simulink model "GHV_open_VarialbeMass_toolbox_adaptive_fuzzy"  (R2023b)
settings: Solver=VariableStepAuto  StartTime=0.0  StopTime=130  FixedStep=0.0000001  MaxStep=0.001  RelTol=1e-3
InitFcn:
  | run('init.m')
undefined symbols (not defined in the file): GHV_cfg
libraries: aerolibasang x3, simulink_extras x2, shared6dof x1, aerolibadyn x1, aerolibatmos2 x1
settings Model: SimulationMode=accelerator  Creator=Admin  LastModifiedBy=Admin
settings SolverCC: AllowMultiTaskInputOutput=on  ZeroCrossControl=EnableAll  ZeroCrossAlgorithm=Adaptive  AutoInsertRateTranBlk=on
settings DebuggingCC: MaskedZcDiagnostic=none  IgnoredZcDiagnostic=none

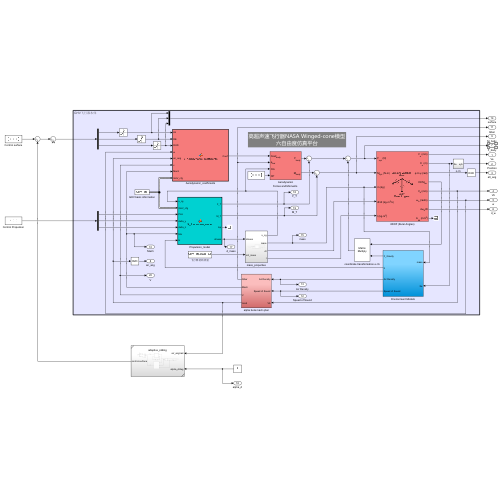
[thumbnail: Simulink's stored preview of the top-level diagram]
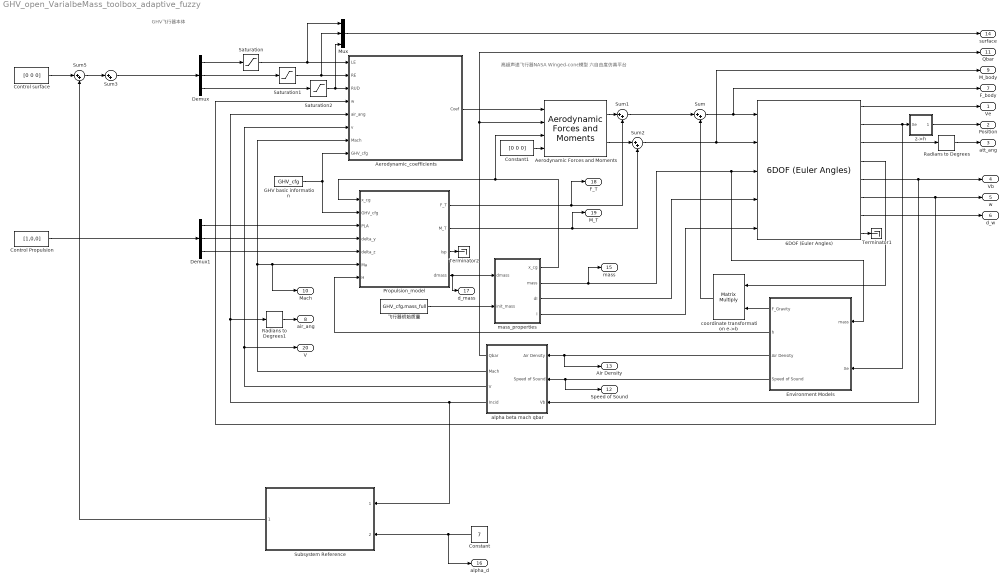
== system GHV_open_VarialbeMass_toolbox_adaptive_fuzzy ==
  note: GHV飞行器本体
  note: 高超声速飞行器NASA Winged-cone模型
      | 六自由度仿真平台
  6DOF (Euler Angles) : shared6dof/6DOF (Euler Angles)  units=Metric (MKS)  mtype=Custom Variable  rep=Euler Angles  xme_0=Position_init  Vm_0=Speed_init  eul_0=Euler_init  pm_0=Omega_init  mass_0=GHV_cfg.mass_full  mass_e=0.5  mass_f=2.0  inertia=GHV_cfg.J  inertia_e=eye(3)  inertia_f=2*eye(3)  k_quat=1.0  vre_flag=off  abi_flag=off  aMode=0  xme_statename=''  Vm_statename=''  eul_statename=''  quat_statename=''  pm_statename=''  mass_statename=''
  "Aerodynamic Forces and Moments " : aerolibadyn/Aerodynamic Forces and Moments   inputAxes=Body  outputForceAxes=Body  outputMomentAxes=Body  S=GHV_cfg.s_ref  b=GHV_cfg.b_ref  cbar=GHV_cfg.c_ref
  Aerodynamic_coefficients : MATLAB Function  TreatAsAtomicUnit=on
  Constant : Constant  Value=7
  Constant1 : Constant  Value=[0 0 0]
  Control Propulsion : Constant  Value=[1,0,0]
  Control surface : Constant  Value=[0 0 0]
  Demux : Demux  Outputs=3
  Demux1 : Demux  Outputs=3
  Environment Models : Subsystem
  GHV basic information : Constant  Value=GHV_cfg  VectorParams1D=off  OutDataTypeStr=Bus: slBus1
  Mux : Mux  Inputs=3
  Propulsion_model : MATLAB Function  TreatAsAtomicUnit=on
  Radians to Degrees : simulink_extras/Transformations/Radians to Degrees
  Radians to Degrees1 : simulink_extras/Transformations/Radians to Degrees
  Saturation : Saturate  UpperLimit=30  LowerLimit=-30
  Saturation1 : Saturate  UpperLimit=30  LowerLimit=-30
  Saturation2 : Saturate  UpperLimit=30  LowerLimit=-30
  Subsystem Reference : Subsystem  ReferencedSubsystem=adaptive_sliding
  Sum{,1..3,5} (5 alike) : Sum  Inputs=|++
  Terminator1 : Terminator
  Terminator2 : Terminator
  alpha beta mach qbar : Subsystem
  coordinate transformation e->b : Product  Multiplication=Matrix(*)
  mass_properties : Subsystem
  z->h : Subsystem
  飞行器初始质量 : Constant  Value=GHV_cfg.mass_full
  Ve : Outport
  Position : Outport  Port=2
  att_ang : Outport  Port=3
  Vb : Outport  Port=4
  w : Outport  Port=5
  d_w : Outport  Port=6
  F_body : Outport  Port=7
  air_ang : Outport  Port=8
  M_body : Outport  Port=9
  Mach : Outport  Port=10
  Qbar : Outport  Port=11
  Speed of Sound : Outport  Port=12
  Air Density : Outport  Port=13
  surface : Outport  Port=14
  mass : Outport  Port=15
  alpha_d : Outport  Port=16
  d_mass : Outport  Port=17
  F_T : Outport  Port=18
  M_T : Outport  Port=19
  V : Outport  Port=20
  wires:
  "Aerodynamic Forces and Moments "/1 -> Sum1/1
  "Aerodynamic Forces and Moments "/2 -> Sum2/1
  Aerodynamic_coefficients/1(Coef) -> "Aerodynamic Forces and Moments "/1
  Environment Models/1(F_Gravity) -> coordinate transformation e->b/2
  6DOF (Euler Angles)/4 -> coordinate transformation e->b/1
  Sum/1 -> 6DOF (Euler Angles)/1, F_body/1
  coordinate transformation e->b/1 -> Sum/2
  6DOF (Euler Angles)/2 -> z->h/1(Xe), Environment Models/2(Xe)
  Environment Models/4(Speed of Sound) -> Speed of Sound/1, alpha beta mach qbar/2(Speed of Sound)
  Environment Models/3(Air Density) -> Air Density/1, alpha beta mach qbar/1(Air Density)
  6DOF (Euler Angles)/5 -> Vb/1, alpha beta mach qbar/3(Vb)
  alpha beta mach qbar/1(Qbar) -> Qbar/1, "Aerodynamic Forces and Moments "/2
  alpha beta mach qbar/4(Incid) -> Subsystem Reference/1, Aerodynamic_coefficients/5(air_ang), Radians to Degrees1/1
  alpha beta mach qbar/3(V) -> V/1, Aerodynamic_coefficients/6(v)
  alpha beta mach qbar/2(Mach) -> Propulsion_model/6(Ma), Mach/1, Aerodynamic_coefficients/7(Mach)
  Constant1/1 -> "Aerodynamic Forces and Moments "/4
  6DOF (Euler Angles)/1 -> Ve/1
  6DOF (Euler Angles)/3 -> Radians to Degrees/1
  6DOF (Euler Angles)/7 -> d_w/1
  6DOF (Euler Angles)/8 -> Terminator1/1
  Control surface/1 -> Sum5/1
  GHV basic information/1 -> Propulsion_model/2(GHV_cfg), Aerodynamic_coefficients/8(GHV_cfg)
  z->h/1(xyh) -> Position/1
  Radians to Degrees/1 -> att_ang/1
  Radians to Degrees1/1 -> air_ang/1
  Demux/3 -> Saturation2/1
  6DOF (Euler Angles)/6 -> w/1, Aerodynamic_coefficients/4(w)
  Saturation/1 -> Mux/1, Aerodynamic_coefficients/1(LE)
  Saturation1/1 -> Mux/2, Aerodynamic_coefficients/2(RE)
  Saturation2/1 -> Mux/3, Aerodynamic_coefficients/3(RUD)
  Environment Models/2(h) -> Propulsion_model/7(H)
  Control Propulsion/1 -> Demux1/1
  Demux1/1 -> Propulsion_model/3(PLA)
  Demux1/3 -> Propulsion_model/5(delta_z)
  Demux1/2 -> Propulsion_model/4(delta_y)
  飞行器初始质量/1 -> mass_properties/2(init_mass)
  Propulsion_model/4(dmass) -> mass_properties/1(dmass), d_mass/1
  mass_properties/2(mass) -> mass/1, Environment Models/1(mass), 6DOF (Euler Angles)/3
  mass_properties/3(dI) -> 6DOF (Euler Angles)/4
  mass_properties/4(I) -> 6DOF (Euler Angles)/5
  mass_properties/1(x_cg) -> Propulsion_model/1(x_cg), "Aerodynamic Forces and Moments "/3
  Sum1/1 -> Sum/1
  Sum2/1 -> 6DOF (Euler Angles)/2, M_body/1
  Propulsion_model/1(F_T) -> F_T/1, Sum1/2
  Propulsion_model/2(M_T) -> M_T/1, Sum2/2
  Propulsion_model/3(Isp) -> Terminator2/1
  Mux/1 -> surface/1
  Constant/1 -> Subsystem Reference/2, alpha_d/1
  Demux/2 -> Saturation1/1
  Demux/1 -> Saturation/1
  Sum5/1 -> Sum3/1
  Subsystem Reference/1 -> Sum5/2
  Sum3/1 -> Demux/1

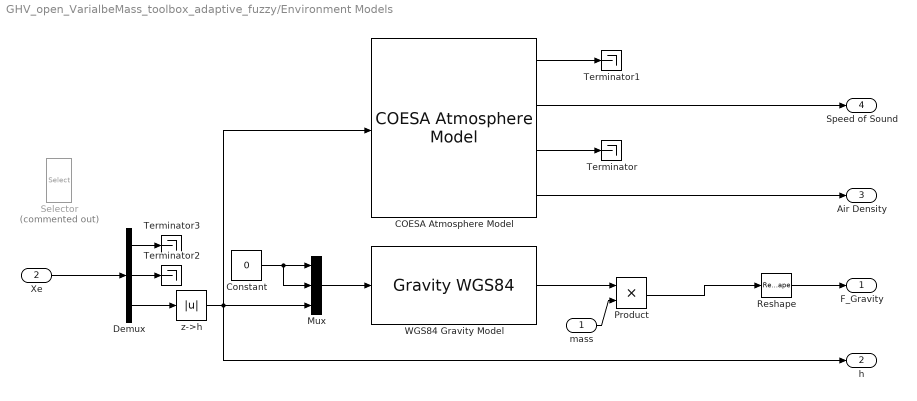
== system GHV_open_VarialbeMass_toolbox_adaptive_fuzzy/Environment Models ==
  mass : Inport
  Xe : Inport  Port=2
  COESA Atmosphere Model : aerolibatmos2/COESA Atmosphere Model  units=Metric (MKS)  spec=1976 COESA-extended U.S. Standard Atmosphere  model=Profile  profile_var=High temperature  profile_percent=1%  profile_alt=5 km (16404 ft)  envelope_var=High temperature  envelope_percent=1%  action=Warning
  Constant : Constant  Value=0
  Demux : Demux  Outputs=3
  Mux : Mux  Inputs=3
  Product : Product
  Reshape : Reshape
  Selector : Selector  Commented=on  InputPortWidth=3  IndexOptions=Index vector (dialog)  Indices=[3]  OutputSizes=1
  Terminator{,1..3} (4 alike) : Terminator
  "WGS84 Gravity Model  " : GravityWGS84  action=None
  z->h : Abs  SaturateOnIntegerOverflow=off
  F_Gravity : Outport
  h : Outport  Port=2
  Air Density : Outport  Port=3
  Speed of Sound : Outport  Port=4
  wires:
  Product/1 -> Reshape/1
  Constant/1 -> Mux/2, Mux/1
  z->h/1 -> h/1, COESA Atmosphere Model/1, Mux/3
  Mux/1 -> "WGS84 Gravity Model  "/1
  COESA Atmosphere Model/1 -> Terminator1/1
  COESA Atmosphere Model/2 -> Speed of Sound/1
  COESA Atmosphere Model/3 -> Terminator/1
  "WGS84 Gravity Model  "/1 -> Product/1
  COESA Atmosphere Model/4 -> Air Density/1
  Reshape/1 -> F_Gravity/1
  Xe/1 -> Demux/1
  Demux/3 -> z->h/1
  Demux/2 -> Terminator2/1
  Demux/1 -> Terminator3/1
  mass/1 -> Product/2

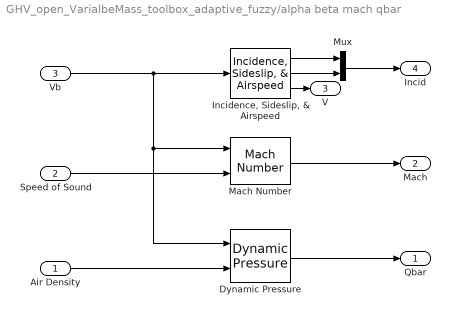
== system GHV_open_VarialbeMass_toolbox_adaptive_fuzzy/alpha beta mach qbar ==
  Air Density : Inport
  Speed of Sound : Inport  Port=2
  Vb : Inport  Port=3
  Dynamic Pressure : aerolibasang/Dynamic Pressure
  "Incidence, Sideslip, & Airspeed" : aerolibasang/Incidence, Sideslip, & Airspeed
  Mach Number : aerolibasang/Mach Number
  Mux : Mux  Inputs=2
  Qbar : Outport
  Mach : Outport  Port=2
  V : Outport  Port=3
  Incid : Outport  Port=4
  wires:
  Speed of Sound/1 -> Mach Number/2
  Mach Number/1 -> Mach/1
  "Incidence, Sideslip, & Airspeed"/2 -> Mux/2
  Vb/1 -> Dynamic Pressure/1, Mach Number/1, "Incidence, Sideslip, & Airspeed"/1
  Dynamic Pressure/1 -> Qbar/1
  Mux/1 -> Incid/1
  "Incidence, Sideslip, & Airspeed"/1 -> Mux/1
  Air Density/1 -> Dynamic Pressure/2
  "Incidence, Sideslip, & Airspeed"/3 -> V/1

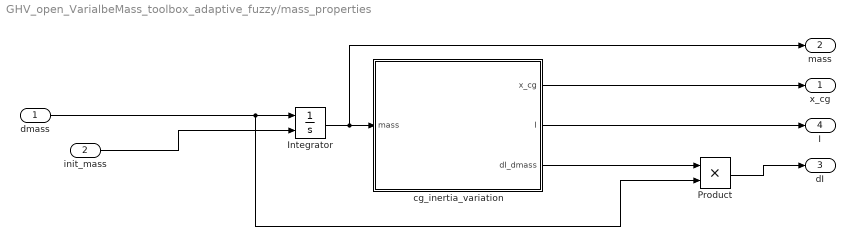
== system GHV_open_VarialbeMass_toolbox_adaptive_fuzzy/mass_properties ==
  dmass : Inport
  init_mass : Inport  Port=2
  Integrator : Integrator  InitialConditionSource=external
  Product : Product
  cg_inertia_variation : MATLAB Function  TreatAsAtomicUnit=on
  x_cg : Outport
  mass : Outport  Port=2
  dI : Outport  Port=3
  I : Outport  Port=4
  wires:
  Integrator/1 -> mass/1, cg_inertia_variation/1(mass)
  init_mass/1 -> Integrator/2
  cg_inertia_variation/3(dI_dmass) -> Product/1
  dmass/1 -> Product/2, Integrator/1
  cg_inertia_variation/2(I) -> I/1
  cg_inertia_variation/1(x_cg) -> x_cg/1
  Product/1 -> dI/1

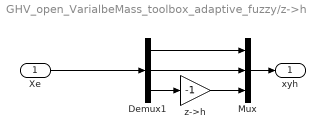
== system GHV_open_VarialbeMass_toolbox_adaptive_fuzzy/z->h ==
  Xe : Inport
  Demux1 : Demux  Outputs=3
  Mux : Mux  Inputs=3
  z->h : Gain  Gain=-1
  xyh : Outport
  wires:
  z->h/1 -> Mux/3
  Demux1/2 -> Mux/2
  Demux1/3 -> z->h/1
  Demux1/1 -> Mux/1
  Xe/1 -> Demux1/1
  Mux/1 -> xyh/1

== matlab function GHV_open_VarialbeMass_toolbox_adaptive_fuzzy/Propulsion_model ==
  data: x_cg input; GHV_cfg input; PLA input; delta_y input; delta_z input; Ma input; H input; F_T output; M_T output; Isp output; dmass output
function  [F_T, M_T, Isp, dmass] = S_Propulsion_model(x_cg, GHV_cfg, PLA, delta_y, delta_z, Ma, H)
    F_T = zeros(3, 1); %#ok<PREALL>
    M_T = zeros(3, 1); %#ok<PREALL>
   [F_T, M_T, Isp, dmass] = Propulsion_model(PLA, H, Ma, delta_y, delta_z, GHV_cfg, x_cg);

end

== matlab function GHV_open_VarialbeMass_toolbox_adaptive_fuzzy/Aerodynamic_coefficients ==
  data: LE input; Coef output; RE input; RUD input; w input; air_ang input; v input; Mach input; GHV_cfg input
function Coef = S_Aerodynamic_coefficients(LE, RE, RUD, w, air_ang,v, Mach, GHV_cfg)
    Coef = zeros(6, 1);
    Coef = Aerodynamic_coefficients(LE, RE, RUD, air_ang, v, w, Mach, GHV_cfg);

end

== matlab function GHV_open_VarialbeMass_toolbox_adaptive_fuzzy/mass_properties/cg_inertia_variation ==
  data: mass input; x_cg output; I output; dI_dmass output
function [x_cg, I, dI_dmass] = S_cg_inertia_variation(mass)

     [x_cg, I, dI_dmass] = cg_inertia_variation(mass);
     
end
